simulink model "FOC_Motor_Control"  (R2020b)
settings: Solver=FixedStepAuto  StartTime=0.0  StopTime=10.0  FixedStep=Fixed_Step_Size  RelTol=1e-3
undefined symbols (not defined in the file): Angle, Angle_offset, atan_table, Cosine_table, Dead_Com_Enable, Dead_Time, DiscIntNeverNeededParam, FF_Enable, Flux, FluxWeak_Enable, FluxWeak_Idref_max, FluxWeak_Idref_min, FluxWeak_Ki, FluxWeak_Kp, Harmonic_Com_Enable, Harmonic_Id5th_Ki, Harmonic_Id5th_Kp, Harmonic_Id5th_Max, Harmonic_Id5th_Min, Harmonic_Id7th_Ki, Harmonic_Id7th_Kp, Harmonic_Id7th_Max, Harmonic_Id7th_Min, Harmonic_Iq5th_Ki, Harmonic_Iq5th_Kp, Harmonic_Iq5th_Max, Harmonic_Iq5th_Min, Harmonic_Iq7th_Ki, Harmonic_Iq7th_Kp, Harmonic_Iq7th_Max, Harmonic_Iq7th_Min, ID_Ki, ID_Kp, inverter, IQ_Ki, IQ_Kp, LADRC_b0, LADRC_Omega_c, Ld, Lq, MTPA_id_table, MTPA_iq_table, MTPA_Te_Max, MTPA_Te_Min, Over_modulation, Pole_Pairs, PWM_Frequency, R, Sine_table, Speed_Ki, Speed_Kp, Speed_PI_OutputMax, Speed_PI_OutputMin, SpeedFilter_Fn, SVPWM, TorqueMode
libraries: simulink x6, powerlib_extras x4, pid_lib x1
(part 2 of 3)

== system FOC_Motor_Control/Motor_Control/Motor_Control_Function/Angle_Speed_100us/Resolver_Observer/Angle_calibration/If Action Subsystem1 ==
  In1 : Inport
  Action Port : ActionPort  ActionPortLabel=else
  Out1 : Outport
  wires:
  In1/1 -> Out1/1

== system FOC_Motor_Control/Motor_Control/Motor_Control_Function/Angle_Speed_100us/Resolver_Observer/Angle_calibration/If Action Subsystem2 ==
  In1 : Inport
  Action Port : ActionPort  ActionPortLabel=if(u1 > 6.283185307)
  2pi : Constant  Value=2*pi  OutDataTypeStr=single
  Subtract1 : Sum  Inputs=+-
  Out1 : Outport
  wires:
  In1/1 -> Subtract1/1
  Subtract1/1 -> Out1/1
  2pi/1 -> Subtract1/2

== system FOC_Motor_Control/Motor_Control/Motor_Control_Function/Angle_Speed_100us/Resolver_Observer/Resolver_Angle_cacl/Sine_Cosine ==
  note: Sine Cosine Coefficients
  P : Inport
  Cosine : Lookup_n-D  NumberOfTableDimensions=1  LookupTableObject=''  BreakpointsForDimension1=[0:2*pi/4095:2*pi]  BreakpointsForDimension1FirstPoint=10  BreakpointsForDimension2FirstPoint=10  BreakpointsForDimension1Spacing=12  BreakpointsForDimension2Spacing=12  IndexSearchMethod=Evenly spaced points  Table=Cosine_table  InterpMethod=Flat  DiagnosticForOutOfRangeInput=Error  InternalRulePriority=Speed  RndMeth=Simplest  InputSameDT=on
  Saturation : Saturate  UpperLimit=2*pi-0.0001  LowerLimit=0+0.0001
  Scope : Scope  NumInputPorts=2
  Sine : Lookup_n-D  NumberOfTableDimensions=1  LookupTableObject=''  BreakpointsForDimension1=[0:2*pi/4095:2*pi]  BreakpointsForDimension1FirstPoint=10  BreakpointsForDimension2FirstPoint=10  BreakpointsForDimension1Spacing=12  BreakpointsForDimension2Spacing=12  IndexSearchMethod=Evenly spaced points  Table=Sine_table  InterpMethod=Flat  DiagnosticForOutOfRangeInput=Error  InternalRulePriority=Speed  RndMeth=Simplest  InputSameDT=on
  Sin : Outport  VectorParamsAs1DForOutWhenUnconnected=off
  Cos : Outport  Port=2  VectorParamsAs1DForOutWhenUnconnected=off
  wires:
  P/1 -> Saturation/1  "position"
  Sine/1 -> Scope/1, Sin/1
  Cosine/1 -> Scope/2, Cos/1
  Saturation/1 -> Cosine/1, Sine/1

== system FOC_Motor_Control/Motor_Control/Motor_Control_Function/Angle_Speed_100us/Speed_Resolver/Speed_cacl/LPF ==
  u : Inport
  Add : Sum  Inputs=+-
  Add1 : Sum
  Constant1 : Constant  Value=SpeedFilter_Fn  OutDataTypeStr=single
  Divide1 : Product  Inputs=**
  Unit Delay : UnitDelay  SampleTime=-1  HasFrameUpgradeWarning=on
  y : Outport
  wires:
  Constant1/1 -> Divide1/1
  u/1 -> Add/1
  Add/1 -> Divide1/2
  Divide1/1 -> Add1/1
  Unit Delay/1 -> Add/2, Add1/2
  Add1/1 -> Unit Delay/1, y/1

== system FOC_Motor_Control/Motor_Control/Motor_Control_Function/Control_Command_2ms/Control_Command_2ms/Speed_PI/SpeedLoop ==
  CMD_RPM : Inport  OutDataTypeStr=single
  FdkRPM : Inport  Port=2  OutDataTypeStr=single
  Reset : Inport  Port=3
  Constant : Constant  Value=LADRC_b0  OutDataTypeStr=single  SampleTime=-1
  Divide : Product  Inputs=*/  OutDataTypeStr=single
  LESO : Subsystem
  Saturation : Saturate  UpperLimit=Speed_PI_OutputMax  LowerLimit=Speed_PI_OutputMin  OutDataTypeStr=single
  Sum : Sum  Inputs=|+-  OutDataTypeStr=single
  Sum1 : Sum  Inputs=|+-  OutDataTypeStr=single
  Unit Delay : UnitDelay  SampleTime=-1  HasFrameUpgradeWarning=on
  omega_c : Gain  Gain=LADRC_Omega_c  OutDataTypeStr=single
  RefIq : Outport  OutDataTypeStr=single
  wires:
  Saturation/1 -> RefIq/1, Unit Delay/1
  Constant/1 -> Divide/2
  Divide/1 -> Saturation/1
  LESO/2(f_hat) -> Sum1/2
  FdkRPM/1 -> LESO/1(FbkSpd)  "FdkRPM"
  LESO/1(omega_r_hat) -> Sum/2
  Sum1/1 -> Divide/1
  omega_c/1 -> Sum1/1
  Sum/1 -> omega_c/1
  CMD_RPM/1 -> Sum/1  "CMD_RPM"
  Unit Delay/1 -> LESO/2(iq)
  Reset/1 -> LESO/3(Reset)

== system FOC_Motor_Control/Motor_Control/Motor_Control_Function/Control_Command_2ms/Control_Command_2ms/Speed_PI/Speed_PI ==
  Ref : Inport
  Fdk : Inport  Port=2
  Reset : Inport  Port=3
  Speed_Control : Subsystem
  Sum : Sum  Inputs=|+-
  PI_out : Outport  VectorParamsAs1DForOutWhenUnconnected=off
  wires:
  Speed_Control/1(PI_Out) -> PI_out/1
  Reset/1 -> Speed_Control/2(Reset)
  Ref/1 -> Sum/1
  Sum/1 -> Speed_Control/1(Err)
  Fdk/1 -> Sum/2

== system FOC_Motor_Control/Motor_Control/Motor_Control_Function/Control_Command_2ms/Flux_weakening /Subsystem/Flux_weak ==
  note: sqrt(Ud*Ud+Uq*Uq)<=Udc/sqrt(3)
  Reset : Inport
  Vd : Inport  Port=2
  Vq : Inport  Port=3
  id_input : Inport  Port=4
  Iq_input : Inport  Port=5
  Bus_voltage : Inport  Port=6
  Add1 : Sum  OutDataTypeStr=Inherit: Same as first input
  Fcn : Fcn  Expr=sqrt(u(1)^2+u(2)^2)
  ID_Control : Subsystem
  If1 : If  IfExpression=u1==1  ElseIfExpressions=u1==0  ShowElse=off
  Merge : Merge
  Mux : Mux  Inputs=2
  Normal : Subsystem  TreatAsAtomicUnit=on
  Over_M : Subsystem  TreatAsAtomicUnit=on
  Over_modulation : Constant  Value=Over_modulation  OutDataTypeStr=boolean
  Sum1 : Sum  Inputs=|-+
  Id_ref : Outport
  iq_ref : Outport  Port=2
  wires:
  Merge/1 -> Sum1/2
  Sum1/1 -> ID_Control/1(Err)
  Mux/1 -> Fcn/1
  Fcn/1 -> Sum1/1
  Vq/1 -> Mux/2
  Iq_input/1 -> iq_ref/1
  id_input/1 -> Add1/1
  Vd/1 -> Mux/1
  Add1/1 -> Id_ref/1
  ID_Control/1(PI_Out) -> Add1/2
  Reset/1 -> ID_Control/2(Reset)
  Bus_voltage/1 -> Normal/1(Bus_voltage), Over_M/1(Bus_voltage)
  Over_modulation/1 -> If1/1
  If1/1 -> Over_M/Action
  If1/2 -> Normal/Action
  Over_M/1(Out1) -> Merge/1
  Normal/1(Out1) -> Merge/2

== system FOC_Motor_Control/Motor_Control/Motor_Control_Function/FOC_Control_100us/FOC/Clarke_Transform/Clark1 ==
  Iabc : Inport
  Add : Sum  Inputs=+--
  Add1 : Sum  Inputs=+-
  Demux : Demux  Outputs=3
  Gain : Gain  Gain=0.5
  Gain1 : Gain  Gain=0.5
  Gain2 : Gain  Gain=sqrt(2/3)
  Gain3 : Gain  Gain=sqrt(3)/2
  Gain4 : Gain  Gain=sqrt(3)/2
  Gain5 : Gain  Gain=sqrt(2/3)
  Ialpha : Outport  VectorParamsAs1DForOutWhenUnconnected=off
  Ibeta : Outport  Port=2  VectorParamsAs1DForOutWhenUnconnected=off
  wires:
  Iabc/1 -> Demux/1
  Demux/1 -> Add/1
  Gain/1 -> Add/2
  Demux/2 -> Gain3/1, Gain/1
  Gain1/1 -> Add/3
  Demux/3 -> Gain4/1, Gain1/1
  Add/1 -> Gain2/1
  Gain2/1 -> Ialpha/1
  Gain3/1 -> Add1/1
  Gain4/1 -> Add1/2
  Add1/1 -> Gain5/1
  Gain5/1 -> Ibeta/1

== system FOC_Motor_Control/Motor_Control/Motor_Control_Function/FOC_Control_100us/FOC/DT_Compensation/DT_Compensation ==
  Ts : Inport
  Td : Inport  Port=2
  Udc : Inport  Port=3
  Id : Inport  Port=4
  Iq : Inport  Port=5
  Theta : Inport  Port=6
  Enable : EnablePort
  Fcn : Fcn  Expr=u(1)*u(3)/u(2)
  IsTheta_Cal : Subsystem
  Mux : Mux  Inputs=3
  Scope : Scope
  Subsystem : Subsystem
  Uabc_alphabeta : Subsystem
  Delta_Ualpha : Outport
  Delta_Ubeta : Outport  Port=2
  wires:
  Udc/1 -> Mux/3
  Ts/1 -> Mux/2
  Td/1 -> Mux/1
  Mux/1 -> Fcn/1
  Fcn/1 -> Subsystem/1(Err_Voltage)
  Id/1 -> IsTheta_Cal/1(Id)
  Iq/1 -> IsTheta_Cal/2(Iq)
  Theta/1 -> IsTheta_Cal/3(d_theta)
  IsTheta_Cal/1(IsTheta) -> Scope/1, Subsystem/2(Istheta)
  Subsystem/1(Uabcc) -> Uabc_alphabeta/1(Uabc)
  Uabc_alphabeta/1(Ualpha) -> Delta_Ualpha/1
  Uabc_alphabeta/2(Ubeta) -> Delta_Ubeta/1

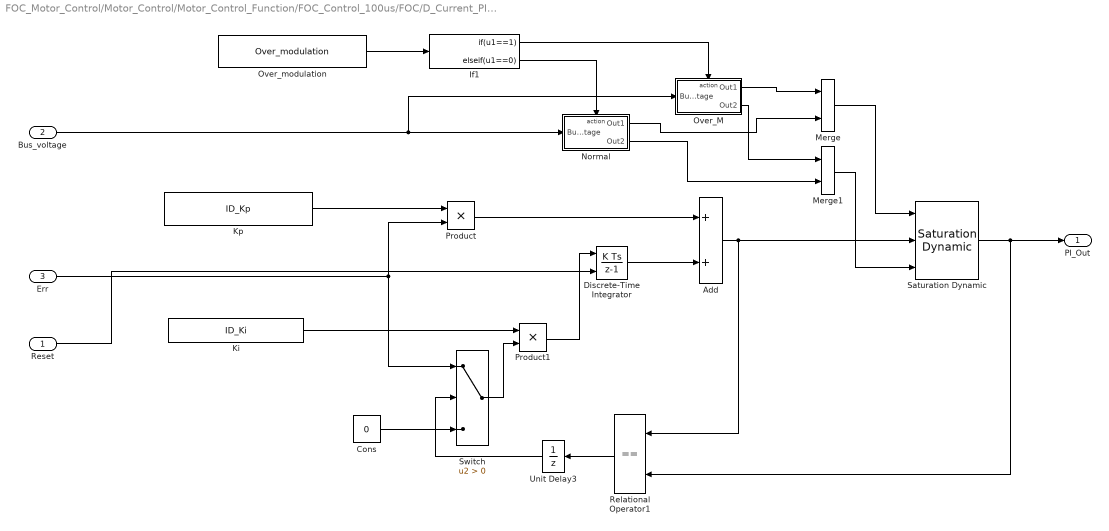
== system FOC_Motor_Control/Motor_Control/Motor_Control_Function/FOC_Control_100us/FOC/D_Current_PI/ID_Control ==
  Reset : Inport
  Bus_voltage : Inport  Port=2
  Err : Inport  Port=3
  Add : Sum
  Cons : Constant  Value=0  OutDataTypeStr=single
  Discrete-Time Integrator : DiscreteIntegrator  ExternalReset=level  SampleTime=-1  ICPrevOutput=DiscIntNeverNeededParam  ICPrevScaledInput=DiscIntNeverNeededParam
  If1 : If  IfExpression=u1==1  ElseIfExpressions=u1==0  ShowElse=off
  Ki : Constant  Value=ID_Ki  OutDataTypeStr=single
  Kp : Constant  Value=ID_Kp  OutDataTypeStr=single
  Merge : Merge
  Merge1 : Merge
  Normal : Subsystem  TreatAsAtomicUnit=on
  Over_M : Subsystem  TreatAsAtomicUnit=on
  Over_modulation : Constant  Value=Over_modulation  OutDataTypeStr=boolean
  Product : Product
  Product1 : Product
  Relational Operator1 : RelationalOperator  Operator===  OutDataTypeStr=boolean  RndMeth=Simplest
  Saturation Dynamic : simulink/Discontinuities/Saturation Dynamic  OutMin=[]  OutMax=[]  OutDataTypeStr=Inherit: Same as second input  OutDataType=fixdt(1, 16)  OutScaling=2^-10  DoSatur=off
  Switch : Switch  Criteria=u2 > Threshold
  Unit Delay3 : UnitDelay  SampleTime=-1  HasFrameUpgradeWarning=on
  PI_Out : Outport
  wires:
  Kp/1 -> Product/1
  Err/1 -> Product/2, Switch/1
  Switch/1 -> Product1/2
  Product1/1 -> Discrete-Time Integrator/1
  Product/1 -> Add/1
  Add/1 -> Saturation Dynamic/2, Relational Operator1/1
  Saturation Dynamic/1 -> Relational Operator1/2, PI_Out/1
  Cons/1 -> Switch/3
  Discrete-Time Integrator/1 -> Add/2
  Relational Operator1/1 -> Unit Delay3/1
  Ki/1 -> Product1/1
  Unit Delay3/1 -> Switch/2
  Reset/1 -> Discrete-Time Integrator/2
  Over_modulation/1 -> If1/1
  If1/2 -> Normal/Action
  If1/1 -> Over_M/Action
  Bus_voltage/1 -> Over_M/1(Bus_voltage), Normal/1(Bus_voltage)
  Over_M/1(Out1) -> Merge/1
  Normal/1(Out1) -> Merge/2
  Over_M/2(Out2) -> Merge1/1
  Normal/2(Out2) -> Merge1/2
  Merge/1 -> Saturation Dynamic/1
  Merge1/1 -> Saturation Dynamic/3

== system FOC_Motor_Control/Motor_Control/Motor_Control_Function/FOC_Control_100us/FOC/FeedForward/Subsystem ==
  note: Vd=id*Rs-we*Lq*iq
  note: Vq=we*Ld*id+iq*Rs+we*flux
  id : Inport
  iq : Inport  Port=2
  we : Inport  Port=3
  Enable : EnablePort
  Ld : Gain  Gain=Ld
  Lq : Gain  Gain=Lq
  Product1 : Product  RndMeth=Zero
  Product2 : Product  RndMeth=Zero
  Rs : Gain  Gain=Rs
  Rs1 : Gain  Gain=Rs
  Subtract1 : Sum  Inputs=+-
  Subtract2 : Sum
  Subtract3 : Sum
  flux : Gain  Gain=flux
  Vd : Outport
  Vq : Outport  Port=2
  wires:
  Subtract2/1 -> Subtract3/1
  Product2/1 -> Subtract2/2
  flux/1 -> Subtract3/2
  Subtract1/1 -> Vd/1
  Rs1/1 -> Subtract2/1
  Ld/1 -> Product2/2
  id/1 -> Rs/1, Product2/1
  iq/1 -> Rs1/1, Product1/2
  Lq/1 -> Product1/1
  Subtract3/1 -> Vq/1
  Rs/1 -> Subtract1/1
  we/1 -> Lq/1, Ld/1, flux/1
  Product1/1 -> Subtract1/2

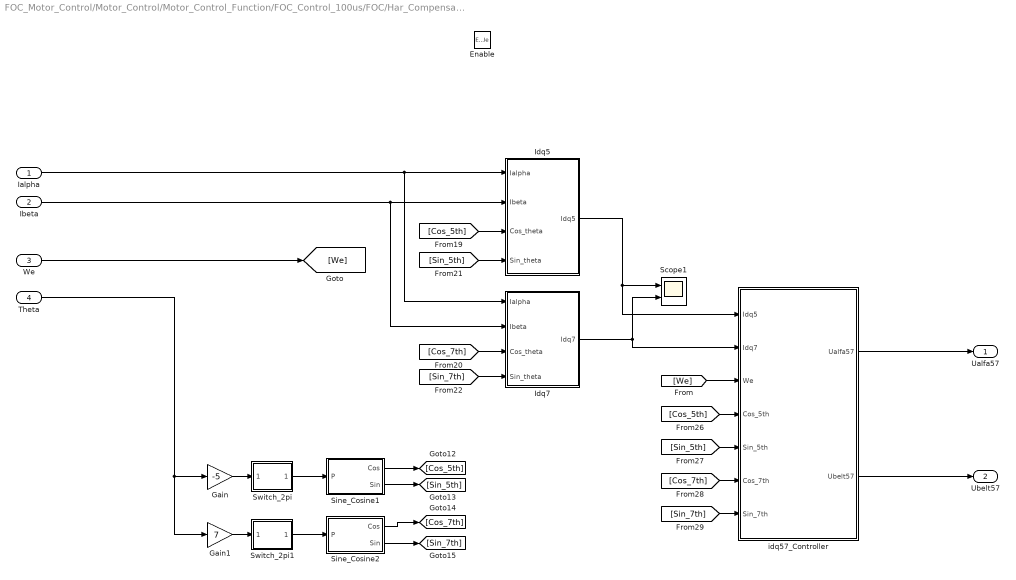
== system FOC_Motor_Control/Motor_Control/Motor_Control_Function/FOC_Control_100us/FOC/Har_Compensation/Har_Compensation ==
  Ialpha : Inport
  Ibeta : Inport  Port=2
  We : Inport  Port=3
  Theta : Inport  Port=4  OutMin=0  OutMax=2*pi
  Enable : EnablePort
  Gain : Gain  Gain=-5
  Gain1 : Gain  Gain=7
  Idq5 : Subsystem
  Idq7 : Subsystem
  Scope1 : Scope  NumInputPorts=2
  Sine_Cosine1 : Subsystem  TreatAsAtomicUnit=on
      settings: RTWSystemCode=Nonreusable function  RTWFcnNameOpts=Use subsystem name
  Sine_Cosine2 : Subsystem  TreatAsAtomicUnit=on
      settings: RTWSystemCode=Nonreusable function  RTWFcnNameOpts=Use subsystem name
  Switch_2pi : Subsystem
  Switch_2pi1 : Subsystem
  idq57_Controller : Subsystem
  Ualfa57 : Outport  VectorParamsAs1DForOutWhenUnconnected=off
  Ubelt57 : Outport  Port=2  VectorParamsAs1DForOutWhenUnconnected=off
  wires:
  idq57_Controller/2(Ubelt57) -> Ubelt57/1
  idq57_Controller/1(Ualfa57) -> Ualfa57/1
  [Cos_5th] -> Idq5/3(Cos_theta)
  [Sin_5th] -> Idq5/4(Sin_theta)
  [Cos_7th] -> idq57_Controller/6(Cos_7th)
  Switch_2pi/1(output) -> Sine_Cosine1/1(P)
  Sine_Cosine1/2(Sin) -> [Sin_5th]
  [Cos_7th] -> Idq7/3(Cos_theta)
  Sine_Cosine2/1(Cos) -> [Cos_7th]
  [Sin_7th] -> idq57_Controller/7(Sin_7th)
  [Sin_5th] -> idq57_Controller/5(Sin_5th)
  Ialpha/1 -> Idq7/1(Ialpha), Idq5/1(Ialpha)
  [Sin_7th] -> Idq7/4(Sin_theta)
  [Cos_5th] -> idq57_Controller/4(Cos_5th)
  Ibeta/1 -> Idq7/2(Ibeta), Idq5/2(Ibeta)
  Switch_2pi1/1(output) -> Sine_Cosine2/1(P)
  Gain1/1 -> Switch_2pi1/1(Input)
  Sine_Cosine2/2(Sin) -> [Sin_7th]
  Gain/1 -> Switch_2pi/1(Input)
  Idq5/1(Idq5) -> idq57_Controller/1(Idq5), Scope1/1
  Sine_Cosine1/1(Cos) -> [Cos_5th]
  Idq7/1(Idq7) -> Scope1/2, idq57_Controller/2(Idq7)
  Theta/1 -> Gain1/1, Gain/1
  We/1 -> [We]
  [We] -> idq57_Controller/3(We)

== system FOC_Motor_Control/Motor_Control/Motor_Control_Function/FOC_Control_100us/FOC/Inverse_Park_Transform/Harmonic_injection ==
  Input : Inport
  Gain2 : Gain  Gain=20
  Gain3 : Gain  Gain=-5
  Gain4 : Gain  Gain=20
  Gain5 : Gain  Gain=-5
  Gain6 : Gain  Gain=5
  Gain7 : Gain  Gain=7
  Gain8 : Gain  Gain=5
  Gain9 : Gain  Gain=7
  Sum3 : Sum  Inputs=|++
  Sum4 : Sum  Inputs=|++
  Trigonometric Function : Trigonometry  Operator=cos
  Trigonometric Function1 : Trigonometry
  Trigonometric Function2 : Trigonometry  Operator=cos
  Trigonometric Function3 : Trigonometry
  Out1 : Outport
  Out2 : Outport  Port=2
  wires:
  Trigonometric Function1/1 -> Gain4/1
  Trigonometric Function/1 -> Gain2/1
  Gain5/1 -> Trigonometric Function1/1
  Trigonometric Function2/1 -> Gain6/1
  Gain7/1 -> Trigonometric Function2/1
  Gain9/1 -> Trigonometric Function3/1
  Trigonometric Function3/1 -> Gain8/1
  Gain2/1 -> Sum3/1
  Gain3/1 -> Trigonometric Function/1
  Gain4/1 -> Sum4/1
  Gain6/1 -> Sum3/2
  Gain8/1 -> Sum4/2
  Sum3/1 -> Out1/1
  Sum4/1 -> Out2/1
  Input/1 -> Gain9/1, Gain5/1, Gain3/1, Gain7/1

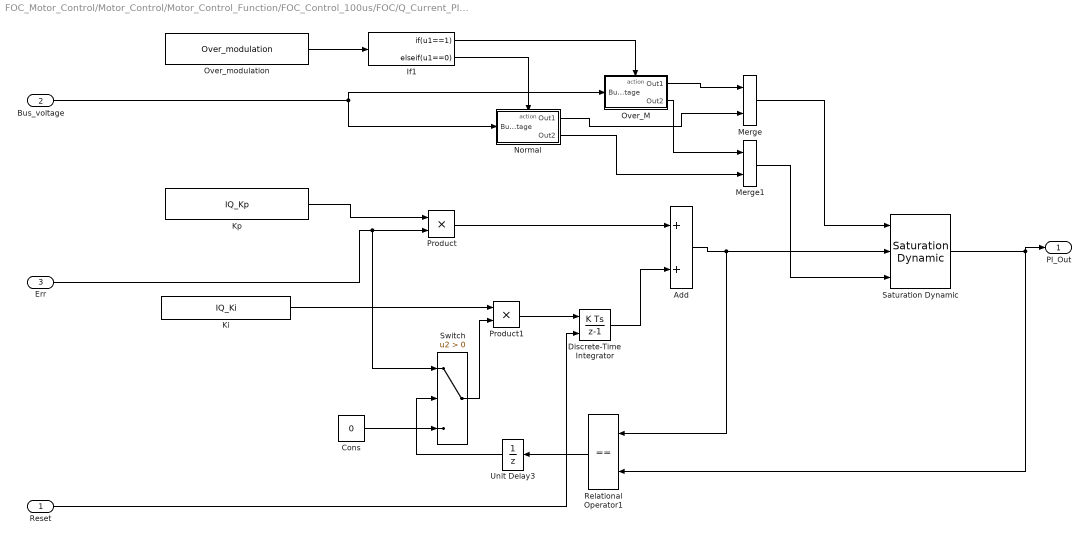
== system FOC_Motor_Control/Motor_Control/Motor_Control_Function/FOC_Control_100us/FOC/Q_Current_PI/IQ_Control ==
  Reset : Inport
  Bus_voltage : Inport  Port=2
  Err : Inport  Port=3
  Add : Sum
  Cons : Constant  Value=0  OutDataTypeStr=single
  Discrete-Time Integrator : DiscreteIntegrator  ExternalReset=level  SampleTime=-1  ICPrevOutput=DiscIntNeverNeededParam  ICPrevScaledInput=DiscIntNeverNeededParam
  If1 : If  IfExpression=u1==1  ElseIfExpressions=u1==0  ShowElse=off
  Ki : Constant  Value=IQ_Ki  OutDataTypeStr=single
  Kp : Constant  Value=IQ_Kp  OutDataTypeStr=single
  Merge : Merge
  Merge1 : Merge
  Normal : Subsystem  TreatAsAtomicUnit=on
  Over_M : Subsystem  TreatAsAtomicUnit=on
  Over_modulation : Constant  Value=Over_modulation  OutDataTypeStr=boolean
  Product : Product
  Product1 : Product
  Relational Operator1 : RelationalOperator  Operator===  OutDataTypeStr=boolean  RndMeth=Simplest
  Saturation Dynamic : simulink/Discontinuities/Saturation Dynamic  OutMin=[]  OutMax=[]  OutDataTypeStr=Inherit: Same as second input  OutDataType=fixdt(1, 16)  OutScaling=2^-10  DoSatur=off
  Switch : Switch  Criteria=u2 > Threshold
  Unit Delay3 : UnitDelay  SampleTime=-1  HasFrameUpgradeWarning=on
  PI_Out : Outport
  wires:
  Kp/1 -> Product/1
  Err/1 -> Switch/1, Product/2
  Switch/1 -> Product1/2
  Product1/1 -> Discrete-Time Integrator/1
  Product/1 -> Add/1
  Add/1 -> Saturation Dynamic/2, Relational Operator1/1
  Saturation Dynamic/1 -> PI_Out/1, Relational Operator1/2
  Cons/1 -> Switch/3
  Discrete-Time Integrator/1 -> Add/2
  Relational Operator1/1 -> Unit Delay3/1
  Ki/1 -> Product1/1
  Unit Delay3/1 -> Switch/2
  Reset/1 -> Discrete-Time Integrator/2
  Normal/1(Out1) -> Merge/2
  Over_M/1(Out1) -> Merge/1
  Over_modulation/1 -> If1/1
  Normal/2(Out2) -> Merge1/2
  If1/2 -> Normal/Action
  Bus_voltage/1 -> Normal/1(Bus_voltage), Over_M/1(Bus_voltage)
  If1/1 -> Over_M/Action
  Over_M/2(Out2) -> Merge1/1
  Merge/1 -> Saturation Dynamic/1
  Merge1/1 -> Saturation Dynamic/3

== system FOC_Motor_Control/Motor_Control/Motor_Control_Function/FOC_Control_100us/FOC/SVPWM/Disable_Motor ==
  Action Port : ActionPort  ActionPortLabel=elseif(u1==1)
  Constant : Constant  Value=0  OutDataTypeStr=single
  Constant1 : Constant  Value=0  OutDataTypeStr=single
  Constant2 : Constant  Value=0  OutDataTypeStr=single
  Out1 : Outport
  Out2 : Outport  Port=2
  Out3 : Outport  Port=3
  wires:
  Constant/1 -> Out1/1
  Constant1/1 -> Out2/1
  Constant2/1 -> Out3/1

== system FOC_Motor_Control/Motor_Control/Motor_Control_Function/FOC_Control_100us/FOC/SVPWM/Enable_Motor ==
  In1 : Inport
  In2 : Inport  Port=2
  In3 : Inport  Port=3
  Action Port : ActionPort  ActionPortLabel=if(u1==0)
  Out1 : Outport
  Out2 : Outport  Port=2
  Out3 : Outport  Port=3
  wires:
  In1/1 -> Out1/1
  In2/1 -> Out2/1
  In3/1 -> Out3/1

== system FOC_Motor_Control/Motor_Control/Motor_Control_Function/FOC_Control_100us/FOC/SVPWM/N Sector  Caculate ==
  Ubelta : Inport
  Ualf : Inport  Port=2
  Add : Sum  Inputs=+++
  Add1 : Sum  Inputs=-+
  Add2 : Sum  Inputs=--
  Constant : Constant  OutDataTypeStr=single
  Constant1 : Constant  Value=0  OutDataTypeStr=single
  Gain : Gain  Gain=sqrt(3)
  Gain1 : Gain  Gain=2
  Gain2 : Gain  Gain=4
  Saturation : Saturate  UpperLimit=6  LowerLimit=1
  Switch : Switch
  Switch1 : Switch
  Switch2 : Switch
  N : Outport
  wires:
  Saturation/1 -> N/1
  Add/1 -> Saturation/1
  Gain2/1 -> Add/3
  Switch2/1 -> Gain2/1
  Add2/1 -> Switch2/2
  Gain1/1 -> Add/2
  Switch1/1 -> Gain1/1
  Add1/1 -> Switch1/2
  Gain/1 -> Add2/2, Add1/2
  Ualf/1 -> Gain/1
  Switch/1 -> Add/1
  Constant1/1 -> Switch/3, Switch1/3, Switch2/3
  Constant/1 -> Switch/1, Switch1/1, Switch2/1
  Ubelta/1 -> Add2/1, Add1/1, Switch/2

== system FOC_Motor_Control/Motor_Control/Motor_Control_Function/FOC_Control_100us/FOC/SVPWM/T1 T2  Caculate ==
  note: Z
  note: Y
  note: -X
  note: X
  note: -Y
  note: Y
  note: -X
  note: X
  note: Z
  note: -Y
  note: -Z
  note: X
  note: Y
  note: Z
  N : Inport
  X : Inport  Port=2
  Y : Inport  Port=3
  Z : Inport  Port=4
  Tpwm : Inport  Port=5
  Add : Sum
  Add1 : Sum  Inputs=-+
  Divide : Product  Inputs=**/
  Divide1 : Product  Inputs=/**
  Gain : Gain  Gain=-1
  Gain1 : Gain  Gain=-1
  Gain2 : Gain  Gain=-1
  Index Vector : MultiPortSwitch  Inputs=6
  Index Vector1 : MultiPortSwitch  Inputs=6
  Switch : Switch  Criteria=u2 > Threshold
  Switch2 : Switch  Criteria=u2 > Threshold
  T1 : Outport
  T2 : Outport  Port=2
  wires:
  Switch2/1 -> T2/1
  Divide1/1 -> Switch2/3
  Switch/1 -> T1/1
  Add1/1 -> Switch/2, Switch2/2
  Add/1 -> Divide1/1, Divide/3, Add1/1
  Tpwm/1 -> Divide1/2, Divide/2, Add1/2
  Divide/1 -> Switch/3
  Index Vector1/1 -> Switch2/1, Add/2, Divide1/3
  Index Vector/1 -> Switch/1, Divide/1, Add/1
  Gain1/1 -> Index Vector/7, Index Vector1/6
  Gain2/1 -> Index Vector/4, Index Vector1/7  "-Z"
  Gain/1 -> Index Vector/5, Index Vector1/3
  Y/1 -> Gain1/1, Index Vector/3, Index Vector1/2
  X/1 -> Index Vector1/4, Index Vector/6, Gain/1
  Z/1 -> Index Vector/2, Index Vector1/5, Gain2/1
  N/1 -> Index Vector1/1, Index Vector/1

== system FOC_Motor_Control/Motor_Control/Motor_Control_Function/FOC_Control_100us/FOC/SVPWM/Tcm calculate ==
  note: Tc
  note: Tb
  note: Ta
  N : Inport
  T1 : Inport  Port=2
  T2 : Inport  Port=3
  Tpwm : Inport  Port=4
  Add : Sum  Inputs=--+
  Add1 : Sum
  Add2 : Sum
  Gain : Gain  Gain=0.5
  Gain1 : Gain  Gain=0.5
  Gain2 : Gain  Gain=1/4
  Index Vector : MultiPortSwitch  Inputs=6
  Index Vector1 : MultiPortSwitch  Inputs=6
  Index Vector2 : MultiPortSwitch  Inputs=6
  Scope2 : Scope  NumInputPorts=3
  Tcm1 : Outport
  Tcm2 : Outport  Port=2
  Tcm3 : Outport  Port=3
  wires:
  Index Vector2/1 -> Scope2/3, Tcm3/1
  N/1 -> Index Vector/1, Index Vector1/1, Index Vector2/1
  Add2/1 -> Index Vector/5, Index Vector/6, Index Vector1/3, Index Vector1/7, Index Vector2/2, Index Vector2/4
  Gain1/1 -> Add2/1
  Add1/1 -> Add2/2, Index Vector/2, Index Vector/7, Index Vector1/4, Index Vector1/5, Index Vector2/3, Index Vector2/6
  Gain2/1 -> Index Vector2/5, Index Vector2/7, Add1/2, Index Vector/3, Index Vector/4, Index Vector1/2, Index Vector1/6
  Gain/1 -> Add1/1
  Add/1 -> Gain2/1
  Tpwm/1 -> Add/3
  T2/1 -> Add/2, Gain1/1
  T1/1 -> Add/1, Gain/1
  Index Vector/1 -> Scope2/1, Tcm1/1
  Index Vector1/1 -> Scope2/2, Tcm2/1

== system FOC_Motor_Control/Motor_Control/Motor_Control_Function/FOC_Control_100us/FOC/SVPWM/XYZ Caculate ==
  note: X
  note: Y
  note: Z
  Ualfpa : Inport
  Ubelta : Inport  Port=2
  Udc : Inport  Port=3
  Tpwm : Inport  Port=4
  Add1 : Sum  Inputs=-+
  Add2 : Sum  Inputs=--
  Constant : Constant  Value=sqrt(3)  OutDataTypeStr=single
  Divide : Product  Inputs=**/
  Gain : Gain  Gain=sqrt(3)
  Gain1 : Gain  Gain=-0.5
  Gain2 : Gain  Gain=-0.5
  Product : Product
  Product1 : Product
  Product2 : Product
  Saturation : Saturate  UpperLimit=1200  LowerLimit=0.0001
  X : Outport
  Y : Outport  Port=2
  Z : Outport  Port=3
  wires:
  Gain2/1 -> Product1/1
  Add2/1 -> Gain2/1
  Add1/1 -> Gain1/1
  Gain/1 -> Add2/2, Add1/2
  Ualfpa/1 -> Gain/1
  Ubelta/1 -> Add2/1, Add1/1, Product/1
  Gain1/1 -> Product2/2
  Product2/1 -> Z/1
  Divide/1 -> Product1/2, Product2/1, Product/2
  Product1/1 -> Y/1
  Product/1 -> X/1
  Udc/1 -> Saturation/1
  Tpwm/1 -> Divide/2
  Constant/1 -> Divide/1
  Saturation/1 -> Divide/3

== system FOC_Motor_Control/Motor_Control/Motor_Control_Function/Control_Command_2ms/Control_Command_2ms/Speed_PI/SpeedLoop/LESO ==
  FbkSpd : Inport  OutDataTypeStr=single  PortDimensions=1
  iq : Inport  Port=2  OutDataTypeStr=single  PortDimensions=1
  Reset : Inport  Port=3
  Constant : Constant  Value=LADRC_Omega_c  OutDataTypeStr=single
  Constant1 : Constant  Value=LADRC_b0  OutDataTypeStr=single  SampleTime=-1
  Discrete-Time Integrator : DiscreteIntegrator  ExternalReset=level  SampleTime=-1  OutDataTypeStr=single  UpperSaturationLimit=6e4  LowerSaturationLimit=-6e4  ICPrevOutput=DiscIntNeverNeededParam  ICPrevScaledInput=DiscIntNeverNeededParam
  Discrete-Time Integrator1 : DiscreteIntegrator  ExternalReset=level  SampleTime=-1  OutDataTypeStr=single  LimitOutput=on  UpperSaturationLimit=2000  LowerSaturationLimit=-2000  ICPrevOutput=DiscIntNeverNeededParam  ICPrevScaledInput=DiscIntNeverNeededParam
  Gain : Gain  Gain=3  OutDataTypeStr=single
  Gain1 : Gain  Gain=2  OutDataTypeStr=single
  Product : Product  Inputs=3  OutDataTypeStr=single
  Product1 : Product  OutDataTypeStr=single
  Product2 : Product  OutDataTypeStr=single
  Sum : Sum  Inputs=|+-  OutDataTypeStr=single
  Sum1 : Sum  Inputs=+++  OutDataTypeStr=single
  omega_r_hat : Outport  OutDataTypeStr=single
  f_hat : Outport  Port=2  OutDataTypeStr=single
  wires:
  Sum/1 -> Gain1/1, Product/3
  Product/1 -> Discrete-Time Integrator/1
  Discrete-Time Integrator/1 -> [f_hat], f_hat/1
  [f_hat] -> Sum1/3
  Sum1/1 -> Discrete-Time Integrator1/1
  Discrete-Time Integrator1/1 -> omega_r_hat/1, [omega_r_hat]
  Product1/1 -> Sum1/1
  FbkSpd/1 -> Sum/1
  [omega_r_hat] -> Sum/2
  Constant/1 -> Gain/1
  Gain1/1 -> Product1/2
  Gain/1 -> Product1/1, Product/2, Product/1
  iq/1 -> Product2/1
  Constant1/1 -> Product2/2
  Product2/1 -> Sum1/2
  Reset/1 -> Discrete-Time Integrator/2, Discrete-Time Integrator1/2

== system FOC_Motor_Control/Motor_Control/Motor_Control_Function/Control_Command_2ms/Control_Command_2ms/Speed_PI/Speed_PI/Speed_Control ==
  Err : Inport
  Reset : Inport  Port=2
  Add : Sum
  Cons : Constant  Value=0  OutDataTypeStr=single
  Discrete-Time Integrator : DiscreteIntegrator  ExternalReset=level  SampleTime=-1  ICPrevOutput=DiscIntNeverNeededParam  ICPrevScaledInput=DiscIntNeverNeededParam
  Ki : Constant  Value=Speed_Ki  OutDataTypeStr=single
  Kp : Constant  Value=Speed_Kp  OutDataTypeStr=single
  Product : Product
  Product1 : Product
  Relational Operator1 : RelationalOperator  Operator===  OutDataTypeStr=boolean  RndMeth=Simplest
  Saturation : Saturate  UpperLimit=Speed_PI_OutputMax  LowerLimit=Speed_PI_OutputMin
  Scope : Scope
  Switch : Switch  Criteria=u2 > Threshold
  Unit Delay3 : UnitDelay  SampleTime=-1  HasFrameUpgradeWarning=on
  PI_Out : Outport
  wires:
  Kp/1 -> Product/1
  Err/1 -> Switch/1, Product/2
  Switch/1 -> Product1/2
  Product1/1 -> Discrete-Time Integrator/1
  Product/1 -> Add/1
  Add/1 -> Relational Operator1/1, Saturation/1
  Saturation/1 -> Relational Operator1/2, PI_Out/1
  Discrete-Time Integrator/1 -> Add/2, Scope/1
  Relational Operator1/1 -> Unit Delay3/1
  Ki/1 -> Product1/1
  Unit Delay3/1 -> Switch/2
  Cons/1 -> Switch/3
  Reset/1 -> Discrete-Time Integrator/2

== system FOC_Motor_Control/Motor_Control/Motor_Control_Function/Control_Command_2ms/Flux_weakening /Subsystem/Flux_weak/ID_Control ==
  Err : Inport
  Reset : Inport  Port=2
  Add : Sum
  Cons : Constant  Value=0  OutDataTypeStr=single
  Discrete-Time Integrator : DiscreteIntegrator  ExternalReset=level  SampleTime=-1  ICPrevOutput=DiscIntNeverNeededParam  ICPrevScaledInput=DiscIntNeverNeededParam
  Ki : Constant  Value=ki  OutDataTypeStr=single
  Kp : Constant  Value=kp  OutDataTypeStr=single
  Product : Product
  Product1 : Product
  Relational Operator1 : RelationalOperator  Operator===  OutDataTypeStr=boolean  RndMeth=Simplest
  Saturation : Saturate  UpperLimit=Id_max  LowerLimit=Id_min
  Switch : Switch  Criteria=u2 > Threshold
  Unit Delay3 : UnitDelay  SampleTime=-1  HasFrameUpgradeWarning=on
  PI_Out : Outport
  wires:
  Kp/1 -> Product/1
  Err/1 -> Switch/1, Product/2
  Switch/1 -> Product1/2
  Product1/1 -> Discrete-Time Integrator/1
  Product/1 -> Add/1
  Add/1 -> Relational Operator1/1, Saturation/1
  Saturation/1 -> Relational Operator1/2, PI_Out/1
  Cons/1 -> Switch/3
  Discrete-Time Integrator/1 -> Add/2
  Relational Operator1/1 -> Unit Delay3/1
  Ki/1 -> Product1/1
  Unit Delay3/1 -> Switch/2
  Reset/1 -> Discrete-Time Integrator/2

== system FOC_Motor_Control/Motor_Control/Motor_Control_Function/Control_Command_2ms/Flux_weakening /Subsystem/Flux_weak/Normal ==
  Bus_voltage : Inport
  Action Port : ActionPort  ActionPortLabel=elseif(u1==0)
  Gain : Gain  Gain=1/sqrt(3)
  Out1 : Outport
  wires:
  Bus_voltage/1 -> Gain/1
  Gain/1 -> Out1/1

== system FOC_Motor_Control/Motor_Control/Motor_Control_Function/Control_Command_2ms/Flux_weakening /Subsystem/Flux_weak/Over_M ==
  Bus_voltage : Inport
  Action Port : ActionPort  ActionPortLabel=if(u1==1)
  Gain : Gain  Gain=2/3
  Out1 : Outport
  wires:
  Bus_voltage/1 -> Gain/1
  Gain/1 -> Out1/1

== system FOC_Motor_Control/Motor_Control/Motor_Control_Function/FOC_Control_100us/FOC/DT_Compensation/DT_Compensation/IsTheta_Cal ==
  Id : Inport
  Iq : Inport  Port=2
  d_theta : Inport  Port=3
  Add1 : Sum
  Angle_calibration : Subsystem
      settings: RTWSystemCode=Nonreusable function  RTWFcnNameOpts=Use subsystem name
  LPF : Subsystem
  LPF1 : Subsystem
  Scope2 : Scope  NumInputPorts=2
  Scope3 : Scope  NumInputPorts=2
  atan : Subsystem
  IsTheta : Outport
  wires:
  d_theta/1 -> Add1/2
  Angle_calibration/1(Angle_output) -> IsTheta/1
  Iq/1 -> LPF/1(u), Scope2/1
  Id/1 -> LPF1/1(u), Scope3/1
  LPF1/1(y) -> [B_Id], Scope3/2
  LPF/1(y) -> Scope2/2, [A_Iq]
  Add1/1 -> Angle_calibration/1(Angle_input)  "Itheta2"
  [A_Iq] -> atan/1(Id)
  [B_Id] -> atan/2(Iq)
  atan/1(Out1) -> Add1/1

== system FOC_Motor_Control/Motor_Control/Motor_Control_Function/FOC_Control_100us/FOC/DT_Compensation/DT_Compensation/Subsystem ==
  Err_Voltage : Inport
  Istheta : Inport  Port=2
  If1 : If  IfExpression=(u1 >5.75958)|(u1<=0.523598)  ElseIfExpressions=(u1 >0.523598)&(u1<=1.570796),(u1 >1.570796)&(u1<=2.617993),(u1 >2.617993)&(u1<=3.665191),(u1 >3.665191)&(u1<=4.7123889),(u1 >4.7123889)&(u1<=5.75958)  ShowElse=off
  Merge : Merge  Inputs=6
  Subsystem : Subsystem
  Subsystem1 : Subsystem
  Subsystem2 : Subsystem
  Subsystem3 : Subsystem
  Subsystem4 : Subsystem
  Subsystem5 : Subsystem
  Uabcc : Outport
  wires:
  Istheta/1 -> If1/1
  If1/1 -> Subsystem/Action
  If1/2 -> Subsystem1/Action
  If1/3 -> Subsystem2/Action
  If1/4 -> Subsystem3/Action
  If1/5 -> Subsystem4/Action
  If1/6 -> Subsystem5/Action
  Err_Voltage/1 -> Subsystem5/1(Voltage), Subsystem3/1(Voltage), Subsystem2/1(Voltage), Subsystem/1(Voltage), Subsystem1/1(Voltage), Subsystem4/1(Voltage)
  Merge/1 -> Uabcc/1
  Subsystem/1(Out1) -> Merge/1
  Subsystem1/1(Out1) -> Merge/2
  Subsystem2/1(Out1) -> Merge/3
  Subsystem3/1(Out1) -> Merge/4
  Subsystem4/1(Out1) -> Merge/5
  Subsystem5/1(Out1) -> Merge/6

== system FOC_Motor_Control/Motor_Control/Motor_Control_Function/FOC_Control_100us/FOC/DT_Compensation/DT_Compensation/Uabc_alphabeta ==
  Uabc : Inport
  Fcn : Fcn  Expr=(2/3)*(u(1)-0.5*u(2)-0.5*u(3))
  Fcn1 : Fcn  Expr=sqrt(1/3)*(u(2)-u(3))
  Ualpha : Outport
  Ubeta : Outport  Port=2
  wires:
  Fcn/1 -> Ualpha/1
  Fcn1/1 -> Ubeta/1
  Uabc/1 -> Fcn1/1, Fcn/1

== system FOC_Motor_Control/Motor_Control/Motor_Control_Function/FOC_Control_100us/FOC/D_Current_PI/ID_Control/Normal ==
  Bus_voltage : Inport
  Action Port : ActionPort  ActionPortLabel=elseif(u1==0)
  Gain : Gain  Gain=1/sqrt(3)
  Gain1 : Gain  Gain=-1/sqrt(3)
  Out1 : Outport
  Out2 : Outport  Port=2
  wires:
  Bus_voltage/1 -> Gain1/1, Gain/1
  Gain/1 -> Out1/1
  Gain1/1 -> Out2/1

== system FOC_Motor_Control/Motor_Control/Motor_Control_Function/FOC_Control_100us/FOC/D_Current_PI/ID_Control/Over_M ==
  Bus_voltage : Inport
  Action Port : ActionPort  ActionPortLabel=if(u1==1)
  Gain : Gain  Gain=2/3
  Gain1 : Gain  Gain=-2/3
  Out1 : Outport
  Out2 : Outport  Port=2
  wires:
  Bus_voltage/1 -> Gain1/1, Gain/1
  Gain/1 -> Out1/1
  Gain1/1 -> Out2/1

== system FOC_Motor_Control/Motor_Control/Motor_Control_Function/FOC_Control_100us/FOC/Har_Compensation/Har_Compensation/Idq5 ==
  Ialpha : Inport
  Ibeta : Inport  Port=2
  Cos_theta : Inport  Port=3
  Sin_theta : Inport  Port=4
  LPF : Subsystem
  LPF2 : Subsystem
  Mux : Mux  Inputs=2
  Park1 : Subsystem
  Scope : Scope  NumInputPorts=2
  Idq5 : Outport  VectorParamsAs1DForOutWhenUnconnected=off
  wires:
  Park1/1(Id5) -> Mux/1
  Park1/2(Iq5) -> Mux/2
  Mux/1 -> Scope/1, LPF/1(u)
  Cos_theta/1 -> Park1/3(Cos_theta)
  Sin_theta/1 -> Park1/4(Sin_theta)
  Ialpha/1 -> Park1/1(Ialf)
  Ibeta/1 -> Park1/2(Ibelt)
  LPF/1(y) -> LPF2/1(u)
  LPF2/1(y) -> Scope/2, Idq5/1

== system FOC_Motor_Control/Motor_Control/Motor_Control_Function/FOC_Control_100us/FOC/Har_Compensation/Har_Compensation/Idq7 ==
  Ialpha : Inport
  Ibeta : Inport  Port=2
  Cos_theta : Inport  Port=3
  Sin_theta : Inport  Port=4
  LPF : Subsystem
  LPF2 : Subsystem
  Mux : Mux  Inputs=2
  Park1 : Subsystem
  Idq7 : Outport  VectorParamsAs1DForOutWhenUnconnected=off
  wires:
  Park1/2(Iq7) -> Mux/2
  Ibeta/1 -> Park1/2(Ibelt)
  Ialpha/1 -> Park1/1(Ialf)
  Park1/1(Id7) -> Mux/1
  Mux/1 -> LPF/1(u)
  Sin_theta/1 -> Park1/4(Sin_theta)
  Cos_theta/1 -> Park1/3(Cos_theta)
  LPF/1(y) -> LPF2/1(u)
  LPF2/1(y) -> Idq7/1

== system FOC_Motor_Control/Motor_Control/Motor_Control_Function/FOC_Control_100us/FOC/Har_Compensation/Har_Compensation/Sine_Cosine1 ==
  note: Sine Cosine Coefficients
  P : Inport
  Cosine : Lookup_n-D  NumberOfTableDimensions=1  LookupTableObject=''  BreakpointsForDimension1=[0:2*pi/4095:2*pi]  BreakpointsForDimension1FirstPoint=10  BreakpointsForDimension2FirstPoint=10  BreakpointsForDimension1Spacing=12  BreakpointsForDimension2Spacing=12  IndexSearchMethod=Evenly spaced points  Table=Cosine_table  InterpMethod=Flat  DiagnosticForOutOfRangeInput=Error  InternalRulePriority=Speed  RndMeth=Simplest  InputSameDT=on
  Saturation : Saturate  UpperLimit=2*pi-0.0001  LowerLimit=0+0.0001
  Scope : Scope  NumInputPorts=2
  Sine : Lookup_n-D  NumberOfTableDimensions=1  LookupTableObject=''  BreakpointsForDimension1=[0:2*pi/4095:2*pi]  BreakpointsForDimension1FirstPoint=10  BreakpointsForDimension2FirstPoint=10  BreakpointsForDimension1Spacing=12  BreakpointsForDimension2Spacing=12  IndexSearchMethod=Evenly spaced points  Table=Sine_table  InterpMethod=Flat  DiagnosticForOutOfRangeInput=Error  InternalRulePriority=Speed  RndMeth=Simplest  InputSameDT=on
  Cos : Outport  VectorParamsAs1DForOutWhenUnconnected=off
  Sin : Outport  Port=2  VectorParamsAs1DForOutWhenUnconnected=off
  wires:
  P/1 -> Saturation/1  "position"
  Sine/1 -> Scope/1, Sin/1
  Cosine/1 -> Scope/2, Cos/1
  Saturation/1 -> Cosine/1, Sine/1

== system FOC_Motor_Control/Motor_Control/Motor_Control_Function/FOC_Control_100us/FOC/Har_Compensation/Har_Compensation/Sine_Cosine2 ==
  note: Sine Cosine Coefficients
  P : Inport
  Cosine : Lookup_n-D  NumberOfTableDimensions=1  LookupTableObject=''  BreakpointsForDimension1=[0:2*pi/4095:2*pi]  BreakpointsForDimension1FirstPoint=10  BreakpointsForDimension2FirstPoint=10  BreakpointsForDimension1Spacing=12  BreakpointsForDimension2Spacing=12  IndexSearchMethod=Evenly spaced points  Table=Cosine_table  InterpMethod=Flat  DiagnosticForOutOfRangeInput=Error  InternalRulePriority=Speed  RndMeth=Simplest  InputSameDT=on
  Saturation : Saturate  UpperLimit=2*pi-0.0001  LowerLimit=0+0.0001
  Scope : Scope  NumInputPorts=2
  Sine : Lookup_n-D  NumberOfTableDimensions=1  LookupTableObject=''  BreakpointsForDimension1=[0:2*pi/4095:2*pi]  BreakpointsForDimension1FirstPoint=10  BreakpointsForDimension2FirstPoint=10  BreakpointsForDimension1Spacing=12  BreakpointsForDimension2Spacing=12  IndexSearchMethod=Evenly spaced points  Table=Sine_table  InterpMethod=Flat  DiagnosticForOutOfRangeInput=Error  InternalRulePriority=Speed  RndMeth=Simplest  InputSameDT=on
  Cos : Outport  VectorParamsAs1DForOutWhenUnconnected=off
  Sin : Outport  Port=2  VectorParamsAs1DForOutWhenUnconnected=off
  wires:
  P/1 -> Saturation/1  "position"
  Sine/1 -> Scope/1, Sin/1
  Cosine/1 -> Scope/2, Cos/1
  Saturation/1 -> Cosine/1, Sine/1

== system FOC_Motor_Control/Motor_Control/Motor_Control_Function/FOC_Control_100us/FOC/Har_Compensation/Har_Compensation/Switch_2pi ==
  Input : Inport
  Data Type Conversion : DataTypeConversion  OutDataTypeStr=int32
  Divide : Product  Inputs=*/
  Divide1 : Product  Inputs=**
  Subtract : Sum  Inputs=-+
  Te2 : Constant  Value=2*pi  OutDataTypeStr=single
  Te3 : Constant  Value=2*pi  OutDataTypeStr=single
  output : Outport
  wires:
  Te3/1 -> Divide1/2
  Data Type Conversion/1 -> Divide1/1
  Divide/1 -> Data Type Conversion/1
  Divide1/1 -> Subtract/1
  Te2/1 -> Divide/2
  Subtract/1 -> output/1
  Input/1 -> Subtract/2, Divide/1

== system FOC_Motor_Control/Motor_Control/Motor_Control_Function/FOC_Control_100us/FOC/Har_Compensation/Har_Compensation/Switch_2pi1 ==
  Input : Inport
  Data Type Conversion : DataTypeConversion  OutDataTypeStr=int32
  Divide : Product  Inputs=*/
  Divide1 : Product  Inputs=**
  Subtract : Sum  Inputs=-+
  Te2 : Constant  Value=2*pi  OutDataTypeStr=single
  Te3 : Constant  Value=2*pi  OutDataTypeStr=single
  output : Outport
  wires:
  Te3/1 -> Divide1/2
  Data Type Conversion/1 -> Divide1/1
  Divide/1 -> Data Type Conversion/1
  Divide1/1 -> Subtract/1
  Te2/1 -> Divide/2
  Subtract/1 -> output/1
  Input/1 -> Subtract/2, Divide/1

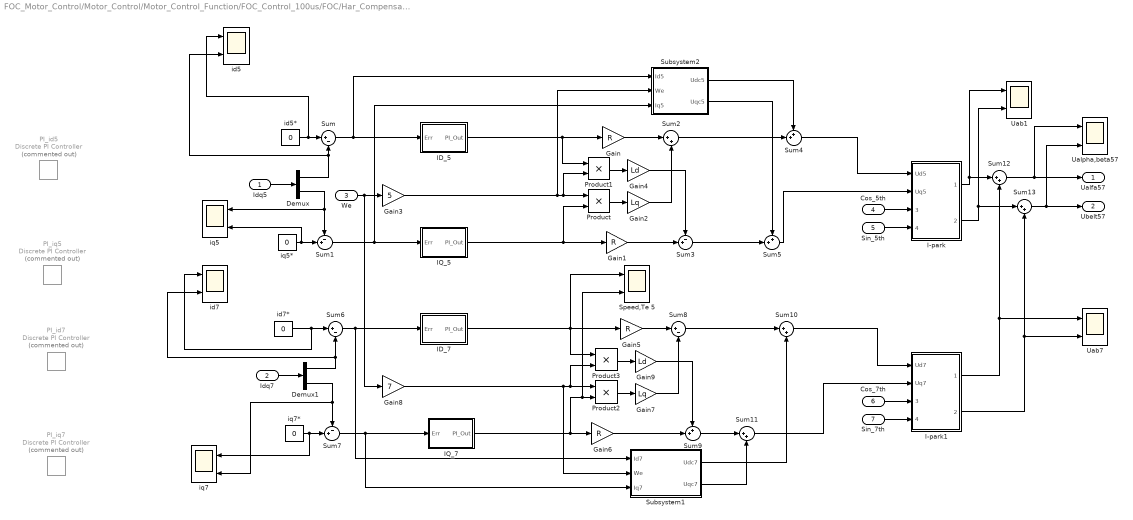
== system FOC_Motor_Control/Motor_Control/Motor_Control_Function/FOC_Control_100us/FOC/Har_Compensation/Har_Compensation/idq57_Controller ==
  Idq5 : Inport
  Idq7 : Inport  Port=2
  We : Inport  Port=3
  Cos_5th : Inport  Port=4
  Sin_5th : Inport  Port=5
  Cos_7th : Inport  Port=6
  Sin_7th : Inport  Port=7
  Demux : Demux  Outputs=2
  Demux1 : Demux  Outputs=2
  Gain{,1,5..6} (4 alike) : Gain  Gain=R
  Gain2 : Gain  Gain=Lq
  Gain3 : Gain  Gain=5
  Gain4 : Gain  Gain=Ld
  Gain7 : Gain  Gain=Lq
  Gain8 : Gain  Gain=7
  Gain9 : Gain  Gain=Ld
  I-park : Subsystem
  I-park1 : Subsystem
  ID_5 : Subsystem
  ID_7 : Subsystem
  IQ_5 : Subsystem
  IQ_7 : Subsystem
  PI_id5 : powerlib_extras/Discrete  Control Blocks/Discrete PI Controller  Commented=on  Kp=Harmonic_Id5th_Kp  Ki=Harmonic_Id5th_Ki  Par_Limits=[60 -60]  Init=0  Ts=-1
  PI_id7 : powerlib_extras/Discrete  Control Blocks/Discrete PI Controller  Commented=on  Kp=Harmonic_Id7th_Kp  Ki=Harmonic_Id7th_Ki  Par_Limits=[60 -60]  Init=0  Ts=-1
  PI_iq5 : powerlib_extras/Discrete  Control Blocks/Discrete PI Controller  Commented=on  Kp=Harmonic_Iq5th_Kp  Ki=Harmonic_Iq5th_Ki  Par_Limits=[60 -60]  Init=0  Ts=-1
  PI_iq7 : powerlib_extras/Discrete  Control Blocks/Discrete PI Controller  Commented=on  Kp=Harmonic_Iq7th_Kp  Ki=Harmonic_Iq7th_Ki  Par_Limits=[60 -60]  Init=0  Ts=-1
  Product{,1..3} (4 alike) : Product
  Speed,Te 5 : Scope  NumInputPorts=2
  Subsystem1 : Subsystem
  Subsystem2 : Subsystem
  Sum : Sum  Inputs=|+-
  Sum1 : Sum  Inputs=-+|
  Sum{2,10..13} (5 alike) : Sum  Inputs=|++
  Sum3 : Sum  Inputs=-+|
  Sum4 : Sum  Inputs=++|
  Sum5 : Sum  Inputs=++|
  Sum6 : Sum  Inputs=|+-
  Sum7 : Sum  Inputs=-+|
  Sum8 : Sum  Inputs=|+-
  Sum9 : Sum  Inputs=++|
  Uab1 : Scope  NumInputPorts=2
  Uab7 : Scope  NumInputPorts=2
  Ualpha,beta57 : Scope  NumInputPorts=2
  id5 : Scope  NumInputPorts=2
  id5* : Constant  Value=0  OutDataTypeStr=single
  id7 : Scope  NumInputPorts=2
  id7* : Constant  Value=0  OutDataTypeStr=single
  iq5 : Scope  NumInputPorts=2
  iq5* : Constant  Value=0  OutDataTypeStr=single
  iq7 : Scope  NumInputPorts=2
  iq7* : Constant  Value=0  OutDataTypeStr=single
  Ualfa57 : Outport  VectorParamsAs1DForOutWhenUnconnected=off
  Ubelt57 : Outport  Port=2  VectorParamsAs1DForOutWhenUnconnected=off
  wires:
  Idq5/1 -> Demux/1
  id5*/1 -> id5/1, Sum/1
  Demux/1 -> id5/2, Sum/2
  Demux/2 -> Sum1/1, iq5/1
  Sum/1 -> ID_5/1(Err), Subsystem2/1(Id5)
  Sum1/1 -> IQ_5/1(Err), Subsystem2/3(Iq5)
  ID_5/1(PI_Out) -> Gain/1, Product1/1
  IQ_5/1(PI_Out) -> Product/2, Gain1/1
  Gain/1 -> Sum2/1
  Product/1 -> Gain2/1
  Gain2/1 -> Sum2/2
  Gain3/1 -> Subsystem2/2(We), Product/1, Product1/2
  Gain1/1 -> Sum3/2
  Product1/1 -> Gain4/1
  Gain4/1 -> Sum3/1
  Gain9/1 -> Sum9/1
  Product3/1 -> Gain9/1
  Gain6/1 -> Sum9/2
  Gain8/1 -> Subsystem1/2(We), Product3/2, Product2/1
  Gain7/1 -> Sum8/2
  Product2/1 -> Gain7/1
  We/1 -> Gain8/1, Gain3/1
  Gain5/1 -> Sum8/1
  IQ_7/1(PI_Out) -> Gain6/1, Speed,Te 5/2, Product2/2
  ID_7/1(PI_Out) -> Product3/1, Speed,Te 5/1, Gain5/1
  Sum7/1 -> IQ_7/1(Err), Subsystem1/3(Iq7)
  Sum6/1 -> ID_7/1(Err), Subsystem1/1(Id7)
  iq7*/1 -> iq7/1, Sum7/2
  id7*/1 -> id7/1, Sum6/1
  Idq7/1 -> Demux1/1
  I-park/1(Ualfa5) -> Uab1/1, Sum12/1
  I-park/2(Ubelt5) -> Uab1/2, Sum13/1
  Sum13/1 -> Ualpha,beta57/2, Ubelt57/1
  Demux1/1 -> Sum6/2, id7/2
  Sum12/1 -> Ualpha,beta57/1, Ualfa57/1
  Sum2/1 -> Sum4/2
  Sum4/1 -> I-park/1(Ud5)
  Sum3/1 -> Sum5/2
  Sum5/1 -> I-park/2(Uq5)
  Sum8/1 -> Sum10/1
  Sum9/1 -> Sum11/1
  Sum10/1 -> I-park1/1(Ud7)
  Sum11/1 -> I-park1/2(Uq7)
  iq5*/1 -> iq5/2, Sum1/2
  I-park1/2(Ubelt7) -> Uab7/2, Sum13/2
  Demux1/2 -> iq7/2, Sum7/1
  Subsystem2/1(Udc5) -> Sum4/1
  Subsystem2/2(Uqc5) -> Sum5/1
  Subsystem1/1(Udc7) -> Sum10/2
  Subsystem1/2(Uqc7) -> Sum11/2
  I-park1/1(Ualfa7) -> Sum12/2, Uab7/1
  Cos_5th/1 -> I-park/3(Cos_theta)
  Sin_5th/1 -> I-park/4(Sin_theta)
  Cos_7th/1 -> I-park1/3(Cos_theta)
  Sin_7th/1 -> I-park1/4(Sin_theta)

== system FOC_Motor_Control/Motor_Control/Motor_Control_Function/FOC_Control_100us/FOC/Q_Current_PI/IQ_Control/Normal ==
  Bus_voltage : Inport
  Action Port : ActionPort  ActionPortLabel=elseif(u1==0)
  Gain : Gain  Gain=1/sqrt(3)
  Gain1 : Gain  Gain=-1/sqrt(3)
  Out1 : Outport
  Out2 : Outport  Port=2
  wires:
  Bus_voltage/1 -> Gain1/1, Gain/1
  Gain/1 -> Out1/1
  Gain1/1 -> Out2/1

== system FOC_Motor_Control/Motor_Control/Motor_Control_Function/FOC_Control_100us/FOC/Q_Current_PI/IQ_Control/Over_M ==
  Bus_voltage : Inport
  Action Port : ActionPort  ActionPortLabel=if(u1==1)
  Gain : Gain  Gain=2/3
  Gain1 : Gain  Gain=-2/3
  Out1 : Outport
  Out2 : Outport  Port=2
  wires:
  Bus_voltage/1 -> Gain1/1, Gain/1
  Gain/1 -> Out1/1
  Gain1/1 -> Out2/1

== system FOC_Motor_Control/Motor_Control/Motor_Control_Function/FOC_Control_100us/FOC/DT_Compensation/DT_Compensation/IsTheta_Cal/Angle_calibration ==
  Angle_input : Inport
  If Action Subsystem1 : Subsystem  TreatAsAtomicUnit=on
  If Action Subsystem2 : Subsystem  TreatAsAtomicUnit=on
  If1 : If  IfExpression=u1 > 6.283185307
  Merge1 : Merge
  Angle_output : Outport
  wires:
  Merge1/1 -> Angle_output/1
  If1/1 -> If Action Subsystem2/Action
  If1/2 -> If Action Subsystem1/Action
  If Action Subsystem2/1(Out1) -> Merge1/1
  Angle_input/1 -> If Action Subsystem1/1(Angle_input), If Action Subsystem2/1(In1), If1/1
  If Action Subsystem1/1(Out1) -> Merge1/2

== system FOC_Motor_Control/Motor_Control/Motor_Control_Function/FOC_Control_100us/FOC/DT_Compensation/DT_Compensation/IsTheta_Cal/LPF ==
  u : Inport
  Add : Sum  Inputs=+-
  Add1 : Sum
  Constant1 : Constant  Value=0.005  OutDataTypeStr=single
  Divide1 : Product  Inputs=**
  Unit Delay : UnitDelay  SampleTime=-1  HasFrameUpgradeWarning=on
  y : Outport
  wires:
  Constant1/1 -> Divide1/1
  u/1 -> Add/1
  Add/1 -> Divide1/2
  Divide1/1 -> Add1/1
  Unit Delay/1 -> Add/2, Add1/2
  Add1/1 -> Unit Delay/1, y/1

== system FOC_Motor_Control/Motor_Control/Motor_Control_Function/FOC_Control_100us/FOC/DT_Compensation/DT_Compensation/IsTheta_Cal/LPF1 ==
  u : Inport
  Add : Sum  Inputs=+-
  Add1 : Sum
  Constant1 : Constant  Value=0.005  OutDataTypeStr=single
  Divide1 : Product  Inputs=**
  Unit Delay : UnitDelay  SampleTime=-1  HasFrameUpgradeWarning=on
  y : Outport
  wires:
  Constant1/1 -> Divide1/1
  u/1 -> Add/1
  Add/1 -> Divide1/2
  Divide1/1 -> Add1/1
  Unit Delay/1 -> Add/2, Add1/2
  Add1/1 -> Unit Delay/1, y/1

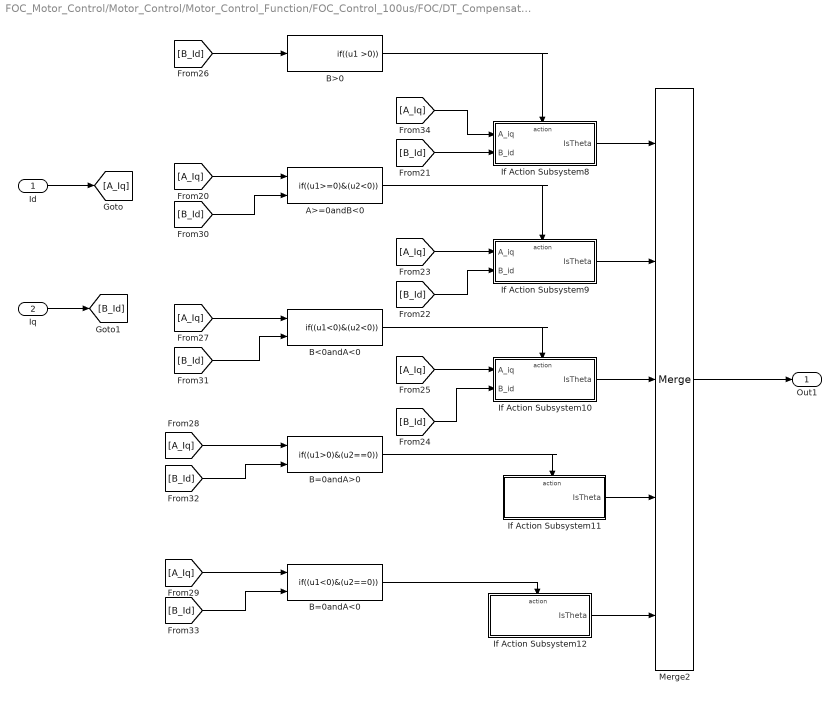
== system FOC_Motor_Control/Motor_Control/Motor_Control_Function/FOC_Control_100us/FOC/DT_Compensation/DT_Compensation/IsTheta_Cal/atan ==
  Id : Inport
  Iq : Inport  Port=2
  A>=0andB<0 : If  NumInputs=2  IfExpression=(u1>=0)&(u2<0)  ShowElse=off
  B<0andA<0 : If  NumInputs=2  IfExpression=(u1<0)&(u2<0)  ShowElse=off
  B=0andA<0 : If  NumInputs=2  IfExpression=(u1<0)&(u2==0)  ShowElse=off
  B=0andA>0 : If  NumInputs=2  IfExpression=(u1>0)&(u2==0)  ShowElse=off
  B>0 : If  IfExpression=(u1 >0)  ShowElse=off
  If Action Subsystem10 : Subsystem  TreatAsAtomicUnit=on
  If Action Subsystem11 : Subsystem  TreatAsAtomicUnit=on
  If Action Subsystem12 : Subsystem  TreatAsAtomicUnit=on
  If Action Subsystem8 : Subsystem  TreatAsAtomicUnit=on
  If Action Subsystem9 : Subsystem  TreatAsAtomicUnit=on
  Merge2 : Merge  Inputs=5
  Out1 : Outport
  wires:
  B<0andA<0/1 -> If Action Subsystem10/Action
  [A_Iq] -> If Action Subsystem10/1(A_iq)
  B=0andA<0/1 -> If Action Subsystem12/Action
  B=0andA>0/1 -> If Action Subsystem11/Action
  [A_Iq] -> If Action Subsystem8/1(A_iq)
  [B_Id] -> B>0/1
  A>=0andB<0/1 -> If Action Subsystem9/Action
  If Action Subsystem11/1(IsTheta) -> Merge2/4
  If Action Subsystem9/1(IsTheta) -> Merge2/2
  [B_Id] -> If Action Subsystem9/2(B_id)
  B>0/1 -> If Action Subsystem8/Action
  [A_Iq] -> If Action Subsystem9/1(A_iq)
  If Action Subsystem8/1(IsTheta) -> Merge2/1
  [B_Id] -> B<0andA<0/2
  [A_Iq] -> A>=0andB<0/1
  [B_Id] -> B=0andA<0/2
  [B_Id] -> A>=0andB<0/2
  [A_Iq] -> B=0andA<0/1
  [A_Iq] -> B=0andA>0/1
  [A_Iq] -> B<0andA<0/1
  [B_Id] -> B=0andA>0/2
  If Action Subsystem12/1(IsTheta) -> Merge2/5
  If Action Subsystem10/1(IsTheta) -> Merge2/3
  Merge2/1 -> Out1/1
  [B_Id] -> If Action Subsystem8/2(B_id)
  [B_Id] -> If Action Subsystem10/2(B_id)
  Id/1 -> [A_Iq]
  Iq/1 -> [B_Id]

== system FOC_Motor_Control/Motor_Control/Motor_Control_Function/FOC_Control_100us/FOC/DT_Compensation/DT_Compensation/Subsystem/Subsystem ==
  Voltage : Inport
  Action Port : ActionPort  ActionPortLabel=if((u1 >5.75958)|(u1<=0.523598))
  Gain : Gain
  Gain1 : Gain  Gain=-1
  Gain2 : Gain  Gain=-1
  Mux1 : Mux  Inputs=3
  Out1 : Outport
  wires:
  Gain/1 -> Mux1/1
  Gain1/1 -> Mux1/2
  Voltage/1 -> Gain2/1, Gain1/1, Gain/1
  Gain2/1 -> Mux1/3
  Mux1/1 -> Out1/1

== system FOC_Motor_Control/Motor_Control/Motor_Control_Function/FOC_Control_100us/FOC/DT_Compensation/DT_Compensation/Subsystem/Subsystem1 ==
  Voltage : Inport
  Action Port : ActionPort  ActionPortLabel=elseif((u1 >0.523598)&(u1<=1.570796))
  Gain : Gain
  Gain1 : Gain
  Gain2 : Gain  Gain=-1
  Mux1 : Mux  Inputs=3
  Out1 : Outport
  wires:
  Mux1/1 -> Out1/1
  Voltage/1 -> Gain2/1, Gain1/1, Gain/1
  Gain/1 -> Mux1/1
  Gain1/1 -> Mux1/2
  Gain2/1 -> Mux1/3

== system FOC_Motor_Control/Motor_Control/Motor_Control_Function/FOC_Control_100us/FOC/DT_Compensation/DT_Compensation/Subsystem/Subsystem2 ==
  Voltage : Inport
  Action Port : ActionPort  ActionPortLabel=elseif((u1 >1.570796)&(u1<=2.617993))
  Gain : Gain  Gain=-1
  Gain1 : Gain
  Gain2 : Gain  Gain=-1
  Mux1 : Mux  Inputs=3
  Out1 : Outport
  wires:
  Mux1/1 -> Out1/1
  Voltage/1 -> Gain2/1, Gain1/1, Gain/1
  Gain/1 -> Mux1/1
  Gain1/1 -> Mux1/2
  Gain2/1 -> Mux1/3

== system FOC_Motor_Control/Motor_Control/Motor_Control_Function/FOC_Control_100us/FOC/DT_Compensation/DT_Compensation/Subsystem/Subsystem3 ==
  Voltage : Inport
  Action Port : ActionPort  ActionPortLabel=elseif((u1 >2.617993)&(u1<=3.665191))
  Gain : Gain  Gain=-1
  Gain1 : Gain
  Gain2 : Gain
  Mux1 : Mux  Inputs=3
  Out1 : Outport
  wires:
  Mux1/1 -> Out1/1
  Voltage/1 -> Gain2/1, Gain1/1, Gain/1
  Gain/1 -> Mux1/1
  Gain1/1 -> Mux1/2
  Gain2/1 -> Mux1/3

== system FOC_Motor_Control/Motor_Control/Motor_Control_Function/FOC_Control_100us/FOC/DT_Compensation/DT_Compensation/Subsystem/Subsystem4 ==
  Voltage : Inport
  Action Port : ActionPort  ActionPortLabel=elseif((u1 >3.665191)&(u1<=4.7123889))
  Gain : Gain  Gain=-1
  Gain1 : Gain  Gain=-1
  Gain2 : Gain
  Mux1 : Mux  Inputs=3
  Out1 : Outport
  wires:
  Mux1/1 -> Out1/1
  Voltage/1 -> Gain2/1, Gain1/1, Gain/1
  Gain/1 -> Mux1/1
  Gain1/1 -> Mux1/2
  Gain2/1 -> Mux1/3

== system FOC_Motor_Control/Motor_Control/Motor_Control_Function/FOC_Control_100us/FOC/DT_Compensation/DT_Compensation/Subsystem/Subsystem5 ==
  Voltage : Inport
  Action Port : ActionPort  ActionPortLabel=elseif((u1 >4.7123889)&(u1<=5.75958))
  Gain : Gain
  Gain1 : Gain  Gain=-1
  Gain2 : Gain
  Mux1 : Mux  Inputs=3
  Out1 : Outport
  wires:
  Mux1/1 -> Out1/1
  Voltage/1 -> Gain2/1, Gain1/1, Gain/1
  Gain/1 -> Mux1/1
  Gain1/1 -> Mux1/2
  Gain2/1 -> Mux1/3

== system FOC_Motor_Control/Motor_Control/Motor_Control_Function/FOC_Control_100us/FOC/Har_Compensation/Har_Compensation/Idq5/LPF ==
  u : Inport
  Add : Sum  Inputs=+-
  Add1 : Sum
  Constant1 : Constant  Value=0.005  OutDataTypeStr=single
  Divide1 : Product  Inputs=**
  Unit Delay : UnitDelay  SampleTime=-1  HasFrameUpgradeWarning=on
  y : Outport
  wires:
  Constant1/1 -> Divide1/1
  u/1 -> Add/1
  Add/1 -> Divide1/2
  Divide1/1 -> Add1/1
  Unit Delay/1 -> Add/2, Add1/2
  Add1/1 -> Unit Delay/1, y/1

== system FOC_Motor_Control/Motor_Control/Motor_Control_Function/FOC_Control_100us/FOC/Har_Compensation/Har_Compensation/Idq5/LPF2 ==
  u : Inport
  Add : Sum  Inputs=+-
  Add1 : Sum
  Constant1 : Constant  Value=0.005  OutDataTypeStr=single
  Divide1 : Product  Inputs=**
  Unit Delay : UnitDelay  SampleTime=-1  HasFrameUpgradeWarning=on
  y : Outport
  wires:
  Constant1/1 -> Divide1/1
  u/1 -> Add/1
  Add/1 -> Divide1/2
  Divide1/1 -> Add1/1
  Unit Delay/1 -> Add/2, Add1/2
  Add1/1 -> Unit Delay/1, y/1

== system FOC_Motor_Control/Motor_Control/Motor_Control_Function/FOC_Control_100us/FOC/Har_Compensation/Har_Compensation/Idq5/Park1 ==
  Ialf : Inport
  Ibelt : Inport  Port=2
  Cos_theta : Inport  Port=3
  Sin_theta : Inport  Port=4
  Fcn2 : Fcn  Expr=u(1)*u(3)+u(2)*u(4)
  Fcn3 : Fcn  Expr=u(2)*u(3)-u(1)*u(4)
  Mux : Mux
  Id5 : Outport  VectorParamsAs1DForOutWhenUnconnected=off
  Iq5 : Outport  Port=2  VectorParamsAs1DForOutWhenUnconnected=off
  wires:
  Fcn3/1 -> Iq5/1
  Fcn2/1 -> Id5/1
  Mux/1 -> Fcn3/1, Fcn2/1
  Sin_theta/1 -> Mux/4
  Cos_theta/1 -> Mux/3
  Ibelt/1 -> Mux/2
  Ialf/1 -> Mux/1

== system FOC_Motor_Control/Motor_Control/Motor_Control_Function/FOC_Control_100us/FOC/Har_Compensation/Har_Compensation/Idq7/LPF ==
  u : Inport
  Add : Sum  Inputs=+-
  Add1 : Sum
  Constant1 : Constant  Value=0.005  OutDataTypeStr=single
  Divide1 : Product  Inputs=**
  Unit Delay : UnitDelay  SampleTime=-1  HasFrameUpgradeWarning=on
  y : Outport
  wires:
  Constant1/1 -> Divide1/1
  u/1 -> Add/1
  Add/1 -> Divide1/2
  Divide1/1 -> Add1/1
  Unit Delay/1 -> Add/2, Add1/2
  Add1/1 -> Unit Delay/1, y/1

== system FOC_Motor_Control/Motor_Control/Motor_Control_Function/FOC_Control_100us/FOC/Har_Compensation/Har_Compensation/Idq7/LPF2 ==
  u : Inport
  Add : Sum  Inputs=+-
  Add1 : Sum
  Constant1 : Constant  Value=0.005  OutDataTypeStr=single
  Divide1 : Product  Inputs=**
  Unit Delay : UnitDelay  SampleTime=-1  HasFrameUpgradeWarning=on
  y : Outport
  wires:
  Constant1/1 -> Divide1/1
  u/1 -> Add/1
  Add/1 -> Divide1/2
  Divide1/1 -> Add1/1
  Unit Delay/1 -> Add/2, Add1/2
  Add1/1 -> Unit Delay/1, y/1

== system FOC_Motor_Control/Motor_Control/Motor_Control_Function/FOC_Control_100us/FOC/Har_Compensation/Har_Compensation/Idq7/Park1 ==
  Ialf : Inport
  Ibelt : Inport  Port=2
  Cos_theta : Inport  Port=3
  Sin_theta : Inport  Port=4
  Fcn2 : Fcn  Expr=u(1)*u(3)+u(2)*u(4)
  Fcn3 : Fcn  Expr=u(2)*u(3)-u(1)*u(4)
  Mux : Mux
  Id7 : Outport  VectorParamsAs1DForOutWhenUnconnected=off
  Iq7 : Outport  Port=2  VectorParamsAs1DForOutWhenUnconnected=off
  wires:
  Ialf/1 -> Mux/1
  Ibelt/1 -> Mux/2
  Cos_theta/1 -> Mux/3
  Sin_theta/1 -> Mux/4
  Mux/1 -> Fcn2/1, Fcn3/1
  Fcn2/1 -> Id7/1
  Fcn3/1 -> Iq7/1

== system FOC_Motor_Control/Motor_Control/Motor_Control_Function/FOC_Control_100us/FOC/Har_Compensation/Har_Compensation/idq57_Controller/I-park ==
  Ud5 : Inport
  Uq5 : Inport  Port=2
  Cos_theta : Inport  Port=3
  Sin_theta : Inport  Port=4
  Fcn : Fcn  Expr=u(1)*u(3)-u(2)*u(4)
  Fcn1 : Fcn  Expr=u(1)*u(4)+u(2)*u(3)
  Mux1 : Mux
  Ualfa5 : Outport  VectorParamsAs1DForOutWhenUnconnected=off
  Ubelt5 : Outport  Port=2  VectorParamsAs1DForOutWhenUnconnected=off
  wires:
  Uq5/1 -> Mux1/2
  Ud5/1 -> Mux1/1
  Fcn1/1 -> Ubelt5/1
  Fcn/1 -> Ualfa5/1
  Mux1/1 -> Fcn1/1, Fcn/1
  Sin_theta/1 -> Mux1/4
  Cos_theta/1 -> Mux1/3
